simulink model "AVR_H2_Hinf__"  (R2022a)
settings: Solver=VariableStepAuto  StartTime=0.0  StopTime=600  RelTol=1e-3
libraries: simulink x1
settings Model: Creator=asus  LastModifiedBy=asus

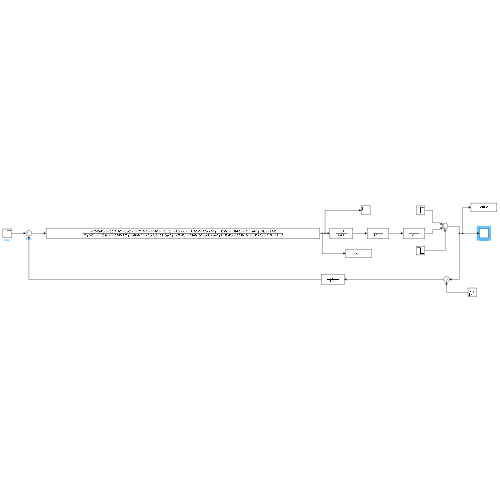
[thumbnail: Simulink's stored preview of the top-level diagram]
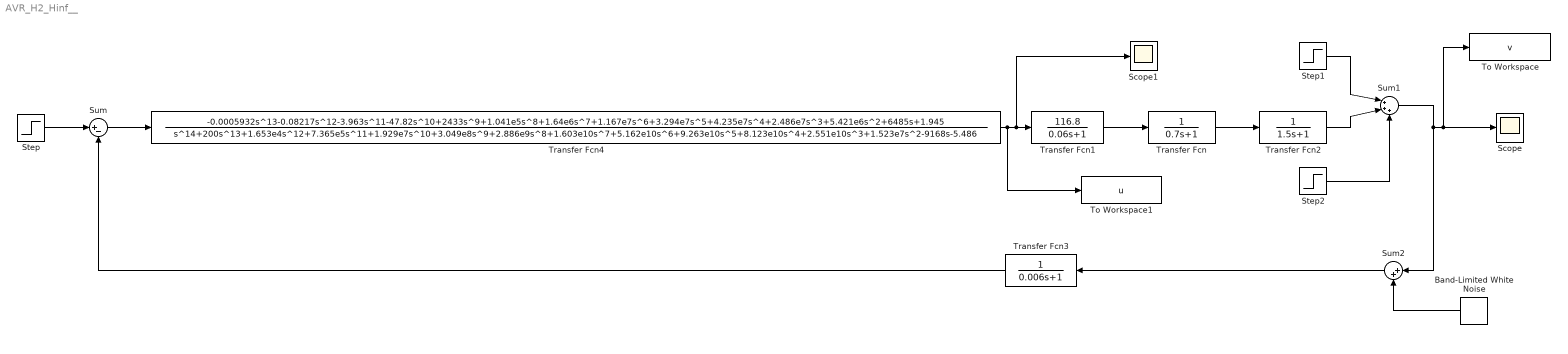
== system AVR_H2_Hinf__ ==
  Band-Limited White Noise : simulink/Sources/Band-Limited White Noise  Cov=[0]  Ts=0.1  seed=[23341]
  Scope : Scope
  Scope1 : Scope
  Step : Step  Time=0  SampleTime=0
  Step1 : Step  Time=200  SampleTime=0
  Step2 : Step  Time=400  After=-1  SampleTime=0
  Sum : Sum  Inputs=|+-
  Sum1 : Sum  Inputs=|+++
  Sum2 : Sum  Inputs=|++
  To Workspace : ToWorkspace  VariableName=v  SaveFormat=Timeseries  SampleTime=-1
  To Workspace1 : ToWorkspace  VariableName=u  SaveFormat=Timeseries  SampleTime=-1
  Transfer Fcn : TransferFcn  Denominator=[0.7 1]
  Transfer Fcn1 : TransferFcn  Numerator=[116.8]  Denominator=[0.06 1]
  Transfer Fcn2 : TransferFcn  Denominator=[1.5 1]
  Transfer Fcn3 : TransferFcn  Denominator=[0.006 1]
  Transfer Fcn4 : TransferFcn  Numerator=[-0.0005932 -0.08217 -3.963 -47.82 2433 1.041e5 1.64e6 1.167e7 3.294e7 4.235e7 2.486e7 5.421e6 6485 1.945]  Denominator=[1 200 1.653e4 7.365e5 1.929e7 3.049e8 2.886e9 1.603e10 5.162e10 9.263e10 8.123e10 2.551e10 1.523e7 -9168 -5.486]
  wires:
  Band-Limited White Noise/1 -> Sum2/2
  Transfer Fcn4/1 -> To Workspace1/1, Scope1/1, Transfer Fcn1/1
  Sum2/1 -> Transfer Fcn3/1
  Step1/1 -> Sum1/1
  Transfer Fcn1/1 -> Transfer Fcn/1
  Step/1 -> Sum/1
  Sum1/1 -> Sum2/1, To Workspace/1, Scope/1
  Step2/1 -> Sum1/3
  Transfer Fcn3/1 -> Sum/2
  Sum/1 -> Transfer Fcn4/1
  Transfer Fcn2/1 -> Sum1/2
  Transfer Fcn/1 -> Transfer Fcn2/1
